simulink model "VoltageSource"  (R2012b)
settings: Solver=ode45  StartTime=0.0  StopTime=10.0  RelTol=1e-3
settings Model: Creator=sz609516  LastModifiedBy=sz609516
settings DataIOCC: SignalLoggingSaveFormat=ModelDataLogs
settings DebuggingCC: FcnCallInpInsideContextMsg=EnableAllAsWarning
settings GRTTargetCC: CombineOutputUpdateFcns=off  GRTInterface=on

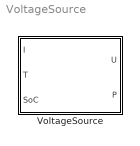
== system VoltageSource ==
  VoltageSource : Subsystem

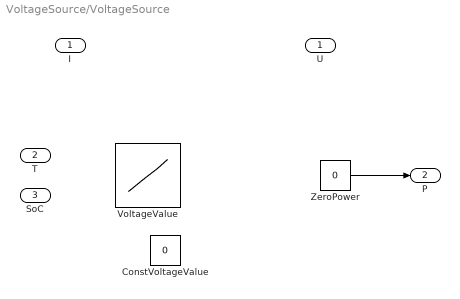
== system VoltageSource/VoltageSource ==
  I : Inport
  T : Inport  Port=2
  SoC : Inport  Port=3
  ConstVoltageValue : Constant  Value=0
  VoltageValue : Lookup_n-D  Table=[1,2,3;4,5,6;7,8,9]  ExtrapMethod=Clip  RndMeth=Simplest  InputSameDT=on
  ZeroPower : Constant  Value=0
  U : Outport
  P : Outport  Port=2
  wires:
  ZeroPower/1 -> P/1
